simulink subsystem "s3s_to_2s"  (R2022b)
settings: Solver=VariableStepAuto  StartTime=0.0  StopTime=10.0  RelTol=1e-3
settings Model: Creator=jack  LastModifiedBy=jack

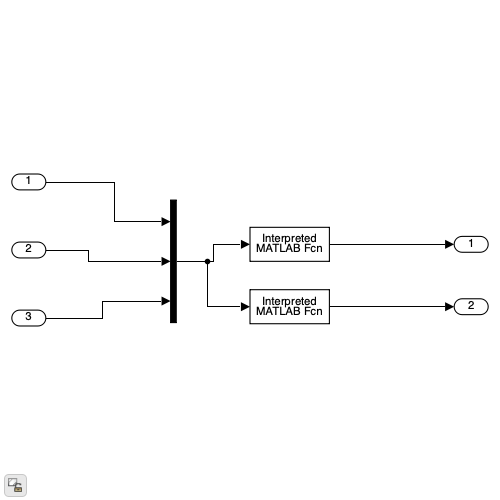
[thumbnail: Simulink's stored preview of the top-level diagram]
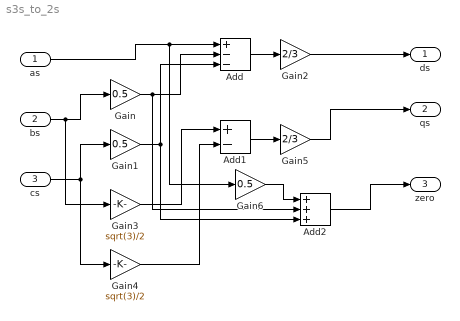
== system s3s_to_2s ==
  as : Inport
  bs : Inport  Port=2
  cs : Inport  Port=3
  Add : Sum  Inputs=+--
  Add1 : Sum  Inputs=+-
  Add2 : Sum  Inputs=+++
  Gain : Gain  Gain=0.5
  Gain1 : Gain  Gain=0.5
  Gain2 : Gain  Gain=2/3
  Gain3 : Gain  Gain=sqrt(3)/2
  Gain4 : Gain  Gain=sqrt(3)/2
  Gain5 : Gain  Gain=2/3
  Gain6 : Gain  Gain=0.5
  ds : Outport
  qs : Outport  Port=2
  zero : Outport  Port=3
  wires:
  as/1 -> Add/1, Gain6/1
  bs/1 -> Gain3/1, Gain/1
  Gain/1 -> Add/2, Add2/2
  cs/1 -> Gain1/1, Gain4/1
  Gain1/1 -> Add/3, Add2/3
  Add/1 -> Gain2/1
  Gain2/1 -> ds/1
  Gain3/1 -> Add1/1
  Gain4/1 -> Add1/2
  Add1/1 -> Gain5/1
  Gain5/1 -> qs/1
  Gain6/1 -> Add2/1
  Add2/1 -> zero/1
